simulink model "Marine_LocoMotive_UAV"  (R2018a)
settings: Solver=ode4  StartTime=0.0  StopTime=60  FixedStep=T  RelTol=1e-3
values from neighbouring files (symbols this model uses):
  a_11 = 0.05*m_b    (= 0.625)    [Marine_LocoMotive_UAV_parameters.m]
  a_33 = m_b    (= 12.5)    [Marine_LocoMotive_UAV_parameters.m]
  A_w = 1*1.5/2    (= 0.75)    [Marine_LocoMotive_UAV_parameters.m]
  A_w2 = 1*0.27/2    (= 0.135)    [Marine_LocoMotive_UAV_parameters.m]
  alpha_bar = pi/4    (= 0.785398163397)    [Marine_LocoMotive_UAV_parameters.m]
  Am = sysd.denominator{1}    [Marine_LocoMotive_UAV_parameters.m]
  Am1_LPF = sysd.denominator{1}    [Marine_LocoMotive_UAV_parameters.m]
  Am2_LPF = sysd.denominator{1}    [Marine_LocoMotive_UAV_parameters.m]
  AmAlpha_LPF = sysd.denominator{1}    [Marine_LocoMotive_UAV_parameters.m]
  AmV_LPF = sysd.denominator{1}    [Marine_LocoMotive_UAV_parameters.m]
  AmZ_LPF = sysd.denominator{1}    [Marine_LocoMotive_UAV_parameters.m]
  b_11 = 0    [Marine_LocoMotive_UAV_parameters.m]
  b_33 = 2*m_b*omega_h    (= 27.5578302946)    [Marine_LocoMotive_UAV_parameters.m]
  Bm = sysd.numerator{1}    [Marine_LocoMotive_UAV_parameters.m]
  Bm1_LPF = sysd.numerator{1}    [Marine_LocoMotive_UAV_parameters.m]
  Bm2_LPF = sysd.numerator{1}    [Marine_LocoMotive_UAV_parameters.m]
  BmAlpha_LPF = sysd.numerator{1}    [Marine_LocoMotive_UAV_parameters.m]
  BmV_LPF = sysd.numerator{1}    [Marine_LocoMotive_UAV_parameters.m]
  BmZ_LPF = sysd.numerator{1}    [Marine_LocoMotive_UAV_parameters.m]
  C_S = [5;9]*10^-3    [Marine_LocoMotive_UAV_parameters.m]
  D_x = b_11 + D_s(1)    [Marine_LocoMotive_UAV_parameters.m]
  D_z = b_33 + D_s(2)    [Marine_LocoMotive_UAV_parameters.m]
  dc_M_p = 6.7    [Marine_LocoMotive_UAV_parameters.m]
  Delta_h = (A_im/A_b-0.5)*h_b    (= -0.0625)    [Marine_LocoMotive_UAV_parameters.m]
  epsilon_1 = 5    [Marine_LocoMotive_UAV_parameters.m]
  epsilon_w = 0    [Marine_LocoMotive_UAV_parameters.m]
  epsilon_w2 = pi    (= 3.14159265359)    [Marine_LocoMotive_UAV_parameters.m]
  g = 9.81    [Marine_LocoMotive_UAV_parameters.m]
  gamma_d_p = 2*0.3/0.03*2*0.2*12/4    (= 24)    [Marine_LocoMotive_UAV_parameters.m]
  H = 10    [Marine_LocoMotive_UAV_parameters.m]
  h_b = 0.25    [Marine_LocoMotive_UAV_parameters.m]
  J_a = m_u*Lc_0^2 + (m_u*(Lc_0/2)^2+m_u*Lc_0/12)    (= 111.3)    [Marine_LocoMotive_UAV_parameters.m]
  J_b = m_b*h_b*l_b/12    (= 0.208333333333)    [Marine_LocoMotive_UAV_parameters.m]
  J_u = 0.03    [Marine_LocoMotive_UAV_parameters.m]
  K = 20    [Marine_LocoMotive_UAV_parameters.m]
  k3 = 4.5    [Marine_LocoMotive_UAV_parameters.m]
  k4 = 2    [Marine_LocoMotive_UAV_parameters.m]
  k_w = omega_w^2/g    (= 0.123862835563)    [Marine_LocoMotive_UAV_parameters.m]
  k_w2 = omega_w2^2/g    (= 0.447144836384)    [Marine_LocoMotive_UAV_parameters.m]
  kd_a = 7    [Marine_LocoMotive_UAV_parameters.m]
  kd_t = 6    [Marine_LocoMotive_UAV_parameters.m]
  kd_T = 0.3    [Marine_LocoMotive_UAV_parameters.m]
  kd_x = 5    [Marine_LocoMotive_UAV_parameters.m]
  kd_z = 2    [Marine_LocoMotive_UAV_parameters.m]
  ki_a = 2    [Marine_LocoMotive_UAV_parameters.m]
  ki_T = 0.8    [Marine_LocoMotive_UAV_parameters.m]
  ki_x = 1.2    [Marine_LocoMotive_UAV_parameters.m]
  ki_z = 1    [Marine_LocoMotive_UAV_parameters.m]
  kp_a = 7    [Marine_LocoMotive_UAV_parameters.m]
  kp_t = 10    [Marine_LocoMotive_UAV_parameters.m]
  kp_T = 5    [Marine_LocoMotive_UAV_parameters.m]
  kp_x = 7    [Marine_LocoMotive_UAV_parameters.m]
  kp_z = 3    [Marine_LocoMotive_UAV_parameters.m]
  L = 0.2    [Marine_LocoMotive_UAV_parameters.m]
  l_b = 0.8    [Marine_LocoMotive_UAV_parameters.m]
  Lc_0 = 7    [Marine_LocoMotive_UAV_parameters.m]
  LIMIT_CMD_PITCH = 45*pi/180    (= 0.785398163397)    [Marine_LocoMotive_UAV_parameters.m]
  LIMIT_uCMD_HEIGHT = 3.5*K    (= 70)    [Marine_LocoMotive_UAV_parameters.m]
  M_a = m_u*Lc_0 + m_c*Lc_0    (= 16.1)    [Marine_LocoMotive_UAV_parameters.m]
  m_b = rho_w*Vol_b/4    (= 12.5)    [Marine_LocoMotive_UAV_parameters.m]
  m_c = 0.5    [Marine_LocoMotive_UAV_parameters.m]
  m_u = 1.8    [Marine_LocoMotive_UAV_parameters.m]
  nu_w = 1.787*10^-6    (= 1.787e-06)    [Marine_LocoMotive_UAV_parameters.m]
  omega_w = 2*pi/T_w    (= 1.10231321179)    [Marine_LocoMotive_UAV_parameters.m]
  omega_w2 = 2*pi/T_w2    (= 2.09439510239)    [Marine_LocoMotive_UAV_parameters.m]
  rho_w = 1000    [Marine_LocoMotive_UAV_parameters.m]
  T = 1/100    (= 0.01)    [Marine_LocoMotive_UAV_parameters.m]
  Theta0 = atan2(V_bar*D_x*cos(alpha_bar_0),V_bar*D_x*sin(alpha_bar_0)+m_u*g*cos(alpha_bar_0))    [Marine_LocoMotive_UAV_parameters.m]
  u_s = w_dir*A_w^2*omega_w*k_w*exp(2*k_w*(-Delta_h/2))    [Marine_LocoMotive_UAV_parameters.m]
  u_s2 = w_dir2*A_w2^2*omega_w2*k_w2*exp(2*k_w2*(-Delta_h/2))    [Marine_LocoMotive_UAV_parameters.m]
  u_t = 0*0.2*1    (= 0)    [Marine_LocoMotive_UAV_parameters.m]
  u_w = 0*0.2    (= 0)    [Marine_LocoMotive_UAV_parameters.m]
  V0_b = [u_t+u_w+u_s+u_s2+v_x_w, v_z_w]    [Marine_LocoMotive_UAV_parameters.m]
  V_bar = 5    [Marine_LocoMotive_UAV_parameters.m]
  Vol_b = A_b*l_b    (= 0.05)    [Marine_LocoMotive_UAV_parameters.m]
  w_dir = 1    [Marine_LocoMotive_UAV_parameters.m]
  w_dir2 = 1    [Marine_LocoMotive_UAV_parameters.m]
  X0_b = [0,H+Zeta_0-Delta_h]    [Marine_LocoMotive_UAV_parameters.m]
  zu_bar = X0_b(2) + Lc_0*sin(alpha_bar_0)    [Marine_LocoMotive_UAV_parameters.m]
undefined symbols (not defined in the file or in its folder): DiscIntNeverNeededParam, k_Da, k_Pa, R_b, Zg
libraries: simulink x30, simulink_extras x3
(part 1 of 3)
settings Model: Creator=Ahmad  LastModifiedBy=Ahmad

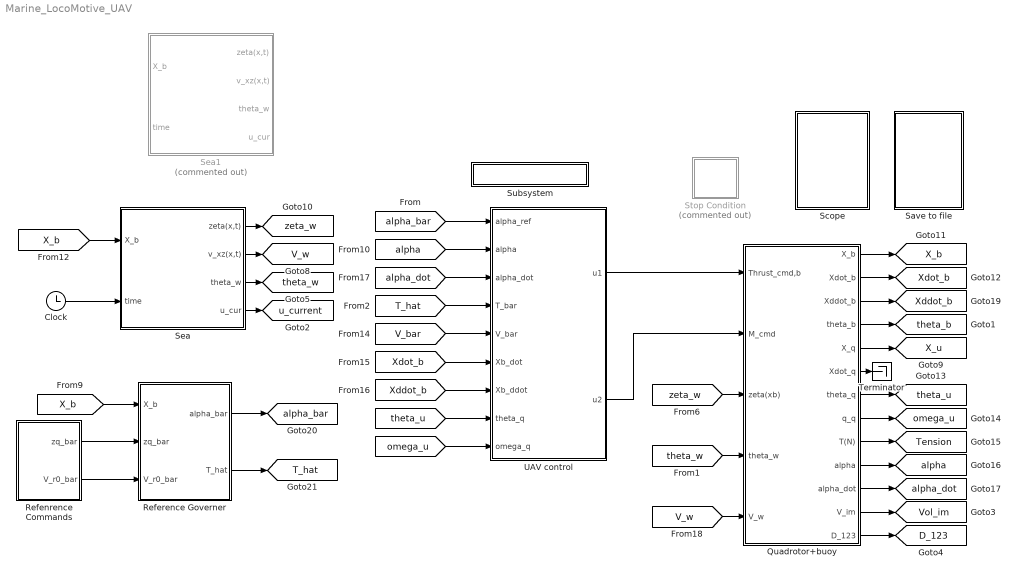
== system Marine_LocoMotive_UAV ==
  Clock : Clock
  Quadrotor+buoy : Subsystem
  Refenrence Commands : Subsystem
  Reference Governer : Subsystem
  Save to file : Subsystem
  Scope : Subsystem
  Sea : Subsystem
  Sea1 : Subsystem  Commented=on
  Stop Condition : Subsystem  Commented=on
  Subsystem : Subsystem
      settings: OpenFcn=Marine_LocoMotive_UAV_parameters
      mask Display:
      | text(.5,.5,'load parameters',...
      | 	'horizontalalignment','center');
  Terminator : Terminator
  UAV control : Subsystem
  tag scope: D_123=global, T_hat=global, Tension=global, V_w=global, Vol_im=global, X_b=global, X_u=global, Xddot_b=global, Xdot_b=global, alpha=global, alpha_bar=global, alpha_dot=global, omega_u=global, theta_b=global, theta_u=global, theta_w=global, u_current=global, zeta_w=global
  wires:
  Clock/1 -> Sea/2(time)
  [X_b] -> Sea/1(X_b)
  Sea/1(zeta(x,t)) -> [zeta_w]
  Sea/2(v_xz(x,t)) -> [V_w]
  Sea/3(theta_w) -> [theta_w]
  [theta_w] -> Quadrotor+buoy/4(theta_w)
  [V_w] -> Quadrotor+buoy/5(V_w)
  [zeta_w] -> Quadrotor+buoy/3(zeta(xb))
  Quadrotor+buoy/5(X_q) -> [X_u]
  Quadrotor+buoy/1(X_b) -> [X_b]
  UAV control/1(u1) -> Quadrotor+buoy/1(Thrust_cmd,b)
  UAV control/2(u2) -> Quadrotor+buoy/2(M_cmd)
  Quadrotor+buoy/2(Xdot_b) -> [Xdot_b]
  Quadrotor+buoy/7(theta_q) -> [theta_u]
  Quadrotor+buoy/8(q_q) -> [omega_u]
  Quadrotor+buoy/9(T(N)) -> [Tension]
  Quadrotor+buoy/10(alpha) -> [alpha]
  Quadrotor+buoy/11(alpha_dot) -> [alpha_dot]
  [X_b] -> Reference Governer/1(X_b)
  Refenrence Commands/1(zq_bar) -> Reference Governer/2(zq_bar)
  Reference Governer/1(alpha_bar) -> [alpha_bar]
  Reference Governer/2(T_hat) -> [T_hat]
  Quadrotor+buoy/3(Xddot_b) -> [Xddot_b]
  Refenrence Commands/2(V_r0_bar) -> Reference Governer/3(V_r0_bar)
  Quadrotor+buoy/4(theta_b) -> [theta_b]
  Quadrotor+buoy/6(Xdot_q) -> Terminator/1
  Sea/4(u_cur) -> [u_current]
  Quadrotor+buoy/12(V_im) -> [Vol_im]
  Quadrotor+buoy/13(D_123) -> [D_123]
  [alpha_bar] -> UAV control/1(alpha_ref)
  [alpha] -> UAV control/2(alpha)
  [alpha_dot] -> UAV control/3(alpha_dot)
  [T_hat] -> UAV control/4(T_bar)
  [V_bar] -> UAV control/5(V_bar)
  [Xdot_b] -> UAV control/6(Xb_dot)
  [Xddot_b] -> UAV control/7(Xb_ddot)
  [theta_u] -> UAV control/8(theta_q)
  [omega_u] -> UAV control/9(omega_q)

== system Marine_LocoMotive_UAV/Quadrotor+buoy ==
  Thrust_cmd,b : Inport
  M_cmd : Inport  Port=2
  zeta(xb) : Inport  Port=3
  theta_w : Inport  Port=4
  V_w : Inport  Port=5
  3-DOF equations of motion Earth frame : Subsystem  mask(3DOF EoM, earth frame){pos_b_ini=X0_b, theta_b_ini=0, alpha_0=alpha_bar, v_b_ini=V0_b, theta_q_ini=Theta0, q_b_ini=0, m_u=m_u, J_u=J_u, m_b=m_b, J_b=J_b, a_ii=[a_11 a_33], b_ii=[D_x,D_z], L=Lc_0, g=g}
      mask prompts: pos_b_ini "Buoy initial position (x z):"; theta_b_ini "Buoy initial body attitude (quadrotor):"; alpha_0 "Cable initial angle:"; v_b_ini "Buoy initial velocity (buoy):"; theta_q_ini "Quadrotor initial body attitude (quadrotor):"; q_b_ini "Quadrotor initial body rotation rate:"; m_u "Quadrotor mass:"; J_u "Quadrotor moment of Inertia:"; m_b "Buoy mass:"; J_b "Buoy moment of Inertia:"; a_ii "Added mass (1x3):"; b_ii "Buoy damping coefficients (1x2):"; L "Cable length:"; g "gravity:"
      mask Display:
      | port_label('input',1,'u_1 (N)','texmode','on');
      | port_label('input',2,'u_2 (N.m)','texmode','on');
      | port_label('input',3,'\zeta (m)','texmode','on');
      | port_label('input',4,'\theta_w (rad)','texmode','on');
      | port_label('input',5,'V_w (N.mm/s)','texmode','on');
      | 
      | port_label('output',1,'X_b (m)','texmode','on');
      | port_label('output',2,'X_{b,dot} (m/s)','texmode','on');
      | port_label('output',3,'X_{b,ddot} (m/s)','texmode','on');
      | port_label('output',4,'\theta_b(rad)','texmode','on');
      | port_label('output',5,'X_q (m)','texmode','on');
      | port_label('output',6,'X_{q,dot} (m/s)','texmode','on');
      | port_label('output',7,'\theta_q(rad)','texmode','on');
      | port_label('output',8,'\omega_q (rad/s)','texmode','on');
      | port_label('output',9,'\alpha (rad)','texmode','on');
      | port_label('output',10,'\alpha_{dot} (rad/s)','texmode','on');
      | port_label('output',11,'T (N)','texmode','on');
      | port_label('output',12,'V_{im} (m^3)','texmode','on');
      | port_label('output',13,'D_{123}','texmode','on');
  Gain : Gain
  Gain1 : Gain
  Mux : Mux  Inputs=2
  Mux1 : Mux  Inputs=2
  Saturation - Limit Height Controller1 : Saturate  UpperLimit=K*L*1.41  LowerLimit=-K*L*1.41
  Saturation - Limit Height Controller3 : Saturate  UpperLimit=4*K  LowerLimit=0
  Torque : Scope
  "Xb " : Scope
  "Xq " : Scope
  motor dynamics (thrust) : DiscreteTransferFcn  Numerator=Bm  Denominator=Am  InitialStates=-Am(2)/Bm(2)*m_u*g/cos(Theta0)
  motor dynamics (torque) : DiscreteTransferFcn  Numerator=Bm  Denominator=Am
  thrust : Scope
  X_b : Outport
  Xdot_b : Outport  Port=2
  Xddot_b : Outport  Port=3
  theta_b : Outport  Port=4
  X_q : Outport  Port=5
  Xdot_q : Outport  Port=6
  theta_q : Outport  Port=7
  q_q : Outport  Port=8
  T(N) : Outport  Port=9
  alpha : Outport  Port=10
  alpha_dot : Outport  Port=11
  V_im : Outport  Port=12
  D_123 : Outport  Port=13
  wires:
  Saturation - Limit Height Controller3/1 -> Gain/1, Mux/2
  motor dynamics (torque)/1 -> Saturation - Limit Height Controller1/1
  M_cmd/1 -> Mux1/1, motor dynamics (torque)/1
  Thrust_cmd,b/1 -> Mux/1, motor dynamics (thrust)/1
  Saturation - Limit Height Controller1/1 -> Mux1/2, Gain1/1
  zeta(xb)/1 -> 3-DOF equations of motion Earth frame/3(zeta)
  theta_w/1 -> 3-DOF equations of motion Earth frame/4(theta_w)
  V_w/1 -> 3-DOF equations of motion Earth frame/5(V_w)
  3-DOF equations of motion Earth frame/5(Xu) -> "Xq "/1, X_q/1  "X_q"
  3-DOF equations of motion Earth frame/1(Xb) -> "Xb "/1, X_b/1  "X_b"
  3-DOF equations of motion Earth frame/2(Xb_dot) -> Xdot_b/1  "Xdot_b"
  3-DOF equations of motion Earth frame/6(Xu_dot) -> Xdot_q/1  "V_q"
  3-DOF equations of motion Earth frame/4(Attitude_buoy) -> theta_b/1  "theta_b"
  3-DOF equations of motion Earth frame/7(Attitude_quadrotor) -> theta_q/1  "theta_q"
  3-DOF equations of motion Earth frame/8(q_quadrotor) -> q_q/1  "omega_q"
  3-DOF equations of motion Earth frame/3(Xb_ddot) -> Xddot_b/1
  motor dynamics (thrust)/1 -> Saturation - Limit Height Controller3/1
  3-DOF equations of motion Earth frame/10(alpha_dot) -> alpha_dot/1  "alpha_dot"
  3-DOF equations of motion Earth frame/11(Cable Tension) -> T(N)/1  "tension"
  3-DOF equations of motion Earth frame/9(alpha) -> alpha/1  "alpha"
  Mux/1 -> thrust/1
  Mux1/1 -> Torque/1
  3-DOF equations of motion Earth frame/12(V_im) -> V_im/1
  Gain/1 -> 3-DOF equations of motion Earth frame/1(u1)
  Gain1/1 -> 3-DOF equations of motion Earth frame/2(u2)
  3-DOF equations of motion Earth frame/13("D_123 ") -> D_123/1

== system Marine_LocoMotive_UAV/Refenrence Commands ==
  note: V_r0_bar is the velocity of the buoy relative
      | to the water current (wave velocity is not included)
  note: Refecence velocity
  "Bias1 " : Bias  Bias=u_t+u_w+u_s
  Bias1 1 : Bias  Commented=on  Bias=u_t+u_w+u_s
  Bias2 : Bias  Bias=-(u_t+u_w+u_s+u_s2)
  Discrete Transfer Fcn : DiscreteTransferFcn  Numerator=BmV_LPF  Denominator=AmV_LPF  InitialStates=sum(AmV_LPF)/sum(BmV_LPF)*0
  Manual Switch : ManualSwitch
  Measured?? (this is not real!) : From  Commented=on  GotoTag=V_w  TagVisibility=global
  Mux : Mux  Inputs=2
  Ramp : simulink/Sources/Ramp  Commented=on  slope=10/40  start=0  InitialOutput=0
  Rate Limiter : RateLimiter  Commented=on  RisingSlewLimit=1/4  FallingSlewLimit=-1/4  SampleTimeMode=inherited
  Step : Step  Time=0  After=V_bar  SampleTime=0
  Step1 : Step  Time=30  After=2  SampleTime=0
  Sum : Sum  Inputs=|+-
  Sum1 : Sum  Inputs=|+-
  V_bar (desired Velocity) : Scope
  v_x : Selector  Commented=on  InputPortWidth=2  IndexOptions=Index vector (dialog)  Indices=[1]  OutputSizes=1
  z_dez : Constant  Value=zu_bar
  zq_bar : Outport
  V_r0_bar : Outport  Port=2
  tag scope: V_bar=global, V_r_bar=global, z_bar=global
  wires:
  Step/1 -> Sum/1
  Step1/1 -> Sum/2
  Measured?? (this is not real!)/1 -> v_x/1
  Manual Switch/1 -> Sum1/2
  Sum1/1 -> V_r0_bar/1, [V_r_bar]  "V_tilde"
  Discrete Transfer Fcn/1 -> "Bias1 "/1
  Mux/1 -> V_bar (desired Velocity)/1
  z_dez/1 -> [z_bar], zq_bar/1
  v_x/1 -> Manual Switch/2
  [u_current] -> Manual Switch/1
  Ramp/1 -> Bias1 1/1
  Bias2/1 -> Discrete Transfer Fcn/1
  Sum/1 -> Bias2/1, Mux/1
  "Bias1 "/1 -> [V_bar], Sum1/1, Mux/2

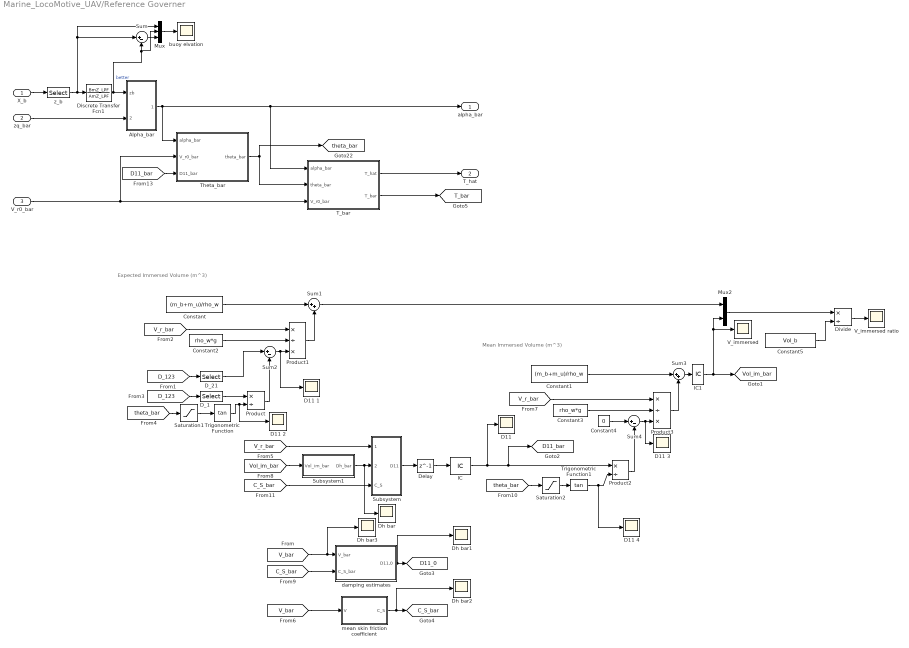
== system Marine_LocoMotive_UAV/Reference Governer ==
  note: Expected Immersed Volume (m^3)
  note: Mean Immersed Volume (m^3)
  X_b : Inport
  zq_bar : Inport  Port=2
  V_r0_bar : Inport  Port=3
  Alpha_bar : Subsystem
  Constant : Constant  Value=(m_b+m_u)/rho_w
  Constant1 : Constant  Value=(m_b+m_u)/rho_w
  Constant2 : Constant  Value=rho_w*g
  Constant3 : Constant  Value=rho_w*g
  Constant4 : Constant  Value=0
  Constant5 : Constant  Value=Vol_b
  D11 {,1..4} (5 alike) : Scope
  D_1 : Selector  NumberOfDimensions=2  InputPortWidth=2  IndexOptions=Index vector (dialog),Index vector (dialog)  Indices=1,1  OutputSizes=1,1
  D_21 : Selector  NumberOfDimensions=2  InputPortWidth=2  IndexOptions=Index vector (dialog),Index vector (dialog)  Indices=2,1  OutputSizes=1,1
  Delay : Delay  DelayLength=1  InitialCondition=0
  Dh bar{,1..3} (4 alike) : Scope
  Discrete Transfer Fcn1 : DiscreteTransferFcn  Numerator=BmZ_LPF  Denominator=AmZ_LPF  InitialStates=[1 1]*(1-sum(AmZ_LPF))/(sum(BmZ_LPF))*X0_b(2)
  Divide : Product  Inputs=*/
  IC : InitialCondition  Value=D_x
  IC1 : InitialCondition  Value=Delta_h*l_b*h_b + l_b*h_b^2/2
  Mux : Mux  Inputs=3
  Mux2 : Mux  Inputs=2
  Product : Product  Inputs=*/
  Product1 : Product  Inputs=*/*
  Product2 : Product  Inputs=*/
  Product3 : Product  Inputs=*/*
  Saturation1 : Saturate  UpperLimit=inf  LowerLimit=0.1*pi/180
  Saturation2 : Saturate  UpperLimit=inf  LowerLimit=0.1*pi/180
  Subsystem : Subsystem
  Subsystem1 : Subsystem
  Sum : Sum  Inputs=|+-
  Sum1 : Sum  Inputs=|++
  Sum2 : Sum  Inputs=|+-
  Sum3 : Sum  Inputs=|++
  Sum4 : Sum  Inputs=|+-
  "T_bar " : Subsystem
  "Theta_bar " : Subsystem
  Trigonometric Function : Trigonometry  Operator=tan
  Trigonometric Function1 : Trigonometry  Operator=tan
  V_immersed : Scope
  V_immersed ratio : Scope
  buoy elvation : Scope
  damping estimates : Subsystem
  "mean skin friction coefficient " : Subsystem
  z_b : Selector  InputPortWidth=2  IndexOptions=Index vector (dialog)  Indices=2  OutputSizes=1
  alpha_bar : Outport
  T_hat : Outport  Port=2
  tag scope: C_S_bar=global, D11_0=global, D11_bar=global, T_bar=global, Vol_im_bar=global, theta_bar=global
  wires:
  X_b/1 -> z_b/1
  "Theta_bar "/1(theta_bar) -> [theta_bar], "T_bar "/2(theta_bar)
  V_r0_bar/1 -> "Theta_bar "/2(V_r0_bar), "T_bar "/3(V_r0_bar)
  zq_bar/1 -> Alpha_bar/2(zq_bar)
  Mux/1 -> buoy elvation/1
  Sum/1 -> Mux/3
  Trigonometric Function/1 -> D11 2/1, Product/2
  Sum1/1 -> Mux2/1
  [theta_bar] -> Saturation1/1
  [D_123] -> D_21/1
  Constant/1 -> Sum1/1
  [V_r_bar] -> Product1/1
  Constant2/1 -> Product1/2
  Product1/1 -> Sum1/2
  Sum2/1 -> D11 1/1, Product1/3
  [D_123] -> D_1/1
  D_21/1 -> Sum2/1
  Product/1 -> Sum2/2
  D_1/1 -> Product/1
  [V_r_bar] -> Subsystem/1(Vr_bar)
  Subsystem1/1(Dh_bar) -> Dh bar/1, Subsystem/2(Dh_bar)
  [Vol_im_bar] -> Subsystem1/1(Vol_im_bar)
  IC/1 -> "D11 "/1, Product2/1, [D11_bar]
  Product2/1 -> Sum4/2
  Constant4/1 -> Sum4/1
  Subsystem/1(D11) -> Delay/1
  Sum4/1 -> D11 3/1, Product3/3
  Product3/1 -> Sum3/2
  Constant3/1 -> Product3/2
  [V_r_bar] -> Product3/1
  Constant1/1 -> Sum3/1
  [theta_bar] -> Saturation2/1
  Trigonometric Function1/1 -> D11 4/1, Product2/2
  Mux2/1 -> Divide/1
  IC1/1 -> V_immersed/1, Mux2/2, [Vol_im_bar]
  Delay/1 -> IC/1
  Sum3/1 -> IC1/1
  Constant5/1 -> Divide/2
  Divide/1 -> V_immersed ratio/1
  z_b/1 -> Discrete Transfer Fcn1/1, Sum/1, Mux/1
  Discrete Transfer Fcn1/1 -> Mux/2, Sum/2, Alpha_bar/1(zb)  "better"
  [V_bar] -> Dh bar3/1, damping estimates/1(V_bar)
  damping estimates/1(D11,0) -> Dh bar1/1, [D11_0]
  [C_S_bar] -> damping estimates/2(C_S_bar)
  [V_bar] -> "mean skin friction coefficient "/1(V)
  [C_S_bar] -> Subsystem/3(C_S)
  "mean skin friction coefficient "/1(C_S) -> Dh bar2/1, [C_S_bar]
  Saturation1/1 -> Trigonometric Function/1
  Saturation2/1 -> Trigonometric Function1/1
  [D11_bar] -> "Theta_bar "/3(D11_bar)
  Alpha_bar/1(alpha_bar) -> alpha_bar/1, "T_bar "/1("alpha_bar "), "Theta_bar "/1("alpha_bar ")
  "T_bar "/1(T_hat) -> T_hat/1
  "T_bar "/2(T_bar) -> [T_bar]

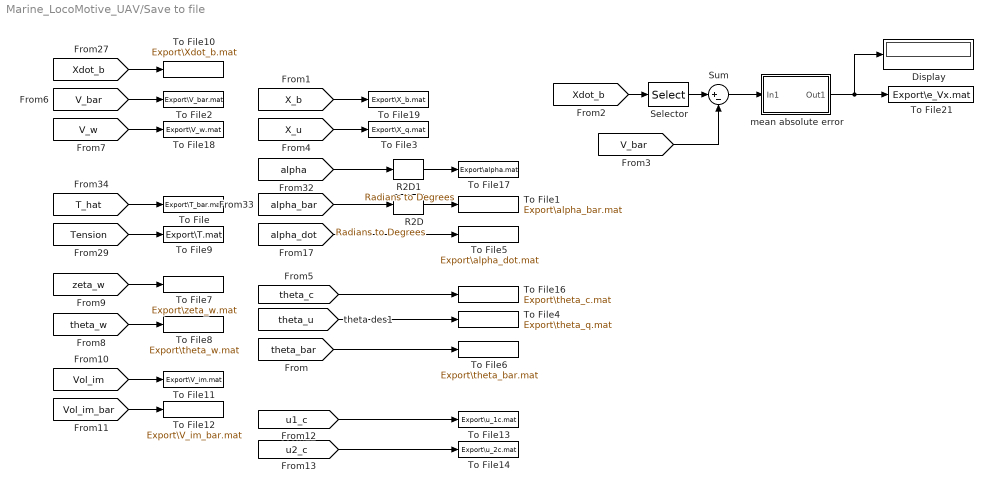
== system Marine_LocoMotive_UAV/Save to file ==
  Display : Display
  R2D : simulink_extras/Transformations/Radians to Degrees
  R2D1 : simulink_extras/Transformations/Radians to Degrees
  Selector : Selector  InputPortWidth=2  IndexOptions=Index vector (dialog)  Indices=1  OutputSizes=1
  Sum : Sum  Inputs=|+-
  To File : ToFile  Filename=Export\T_bar.mat  MatrixName=T_bar  SaveFormat=Timeseries  SampleTime=floor(T/4)
  To File1 : ToFile  Filename=Export\alpha_bar.mat  MatrixName=alpha_bar  SaveFormat=Timeseries  SampleTime=floor(T/4)
  To File10 : ToFile  Filename=Export\Xdot_b.mat  MatrixName=Xdot_b  SaveFormat=Timeseries  SampleTime=floor(T/4)
  To File11 : ToFile  Filename=Export\V_im.mat  MatrixName=V_im  SaveFormat=Timeseries  SampleTime=floor(T/4)
  To File12 : ToFile  Filename=Export\V_im_bar.mat  MatrixName=V_im_bar  SaveFormat=Timeseries  SampleTime=floor(T/4)
  To File13 : ToFile  Filename=Export\u_1c.mat  MatrixName=u_1c  SaveFormat=Timeseries  SampleTime=floor(T/4)
  To File14 : ToFile  Filename=Export\u_2c.mat  MatrixName=u_2c  SaveFormat=Timeseries  SampleTime=floor(T/4)
  To File16 : ToFile  Filename=Export\theta_c.mat  MatrixName=theta_c  SaveFormat=Timeseries  SampleTime=floor(T/4)
  To File17 : ToFile  Filename=Export\alpha.mat  MatrixName=alpha  SaveFormat=Timeseries  SampleTime=floor(T/4)
  To File18 : ToFile  Filename=Export\V_w.mat  MatrixName=V_w  SaveFormat=Timeseries  SampleTime=floor(T/4)
  To File19 : ToFile  Filename=Export\X_b.mat  MatrixName=X_b  SaveFormat=Timeseries  SampleTime=floor(T/4)
  To File2 : ToFile  Filename=Export\V_bar.mat  MatrixName=V_bar  SaveFormat=Timeseries  SampleTime=floor(T/4)
  To File21 : ToFile  Filename=Export\e_Vx.mat  MatrixName=Vx  SaveFormat=Timeseries  SampleTime=floor(T/4)
  To File3 : ToFile  Filename=Export\X_q.mat  MatrixName=X_q  SaveFormat=Timeseries  SampleTime=floor(T/4)
  To File4 : ToFile  Filename=Export\theta_q.mat  MatrixName=theta_q  SaveFormat=Timeseries  SampleTime=floor(T/4)
  To File5 : ToFile  Filename=Export\alpha_dot.mat  MatrixName=alpha_dot  SaveFormat=Timeseries  SampleTime=floor(T/4)
  To File6 : ToFile  Filename=Export\theta_bar.mat  MatrixName=theta_bar  SaveFormat=Timeseries  SampleTime=floor(T/4)
  To File7 : ToFile  Filename=Export\zeta_w.mat  MatrixName=zeta_w  SaveFormat=Timeseries  SampleTime=floor(T/4)
  To File8 : ToFile  Filename=Export\theta_w.mat  MatrixName=theta_w  SaveFormat=Timeseries  SampleTime=floor(T/4)
  To File9 : ToFile  Filename=Export\T.mat  MatrixName=T  SaveFormat=Timeseries  SampleTime=floor(T/4)
  mean absolute error : Subsystem
  wires:
  R2D/1 -> To File1/1
  [X_u] -> To File3/1
  [alpha_bar] -> R2D/1
  [V_bar] -> To File2/1
  [theta_c] -> To File16/1
  [alpha] -> R2D1/1
  R2D1/1 -> To File17/1
  [V_w] -> To File18/1
  [X_b] -> To File19/1
  Sum/1 -> mean absolute error/1(In1)
  mean absolute error/1(Out1) -> Display/1, To File21/1
  [T_hat] -> To File/1
  [theta_u] -> To File4/1
  [alpha_dot] -> To File5/1
  [theta_bar] -> To File6/1
  [zeta_w] -> To File7/1
  [theta_w] -> To File8/1
  [Tension] -> To File9/1
  [Xdot_b] -> To File10/1
  [Xdot_b] -> Selector/1
  [V_bar] -> Sum/2
  Selector/1 -> Sum/1
  [Vol_im] -> To File11/1
  [Vol_im_bar] -> To File12/1
  [u1_c] -> To File13/1
  [u2_c] -> To File14/1

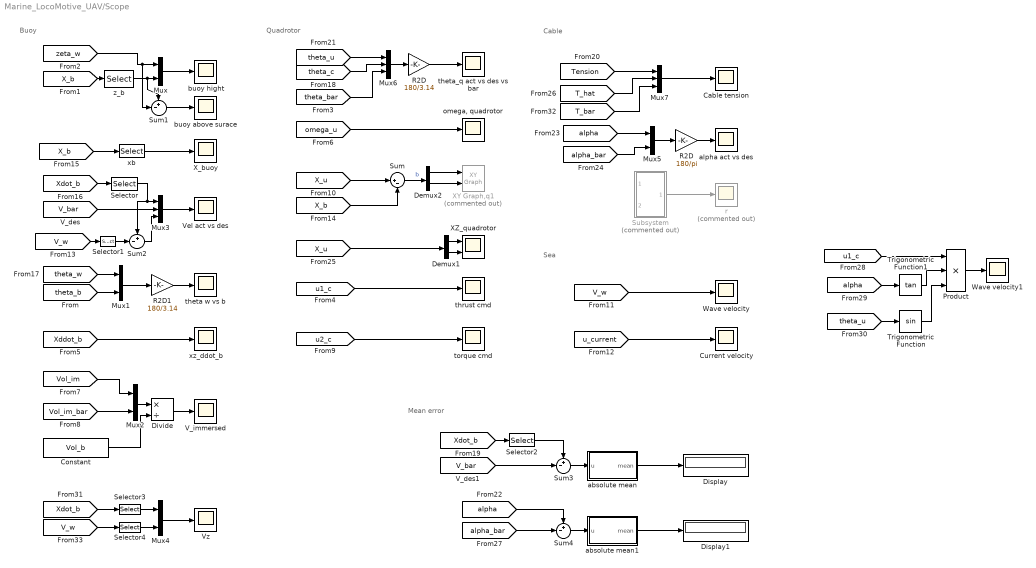
== system Marine_LocoMotive_UAV/Scope ==
  note: Mean error
  note: Sea
  note: Cable
  note: Quadrotor
  note: Buoy
  Cable tension : Scope
  Constant : Constant  Value=Vol_b
  Current velocity : Scope
  Demux1 : Demux  Outputs=2
  Demux2 : Demux  Outputs=2
  Display : Display
  Display1 : Display
  Divide : Product  Inputs=*/
  Mux{,1..2,4..5} (5 alike) : Mux  Inputs=2
  Mux3 : Mux  Inputs=3
  Mux6 : Mux  Inputs=3
  Mux7 : Mux  Inputs=3
  Product : Product  Inputs=3
  R2D : Gain  Gain=180/3.14
  "R2D " : Gain  Gain=180/pi
  R2D1 : Gain  Gain=180/3.14
  Selector : Selector  InputPortWidth=2  IndexOptions=Index vector (dialog)  Indices=1  OutputSizes=1
  Selector1 : Selector  InputPortWidth=2  IndexOptions=Index vector (dialog)  Indices=1  OutputSizes=1
  Selector2 : Selector  InputPortWidth=2  IndexOptions=Index vector (dialog)  Indices=1  OutputSizes=1
  Selector3 : Selector  InputPortWidth=2  IndexOptions=Index vector (dialog)  Indices=2  OutputSizes=1
  Selector4 : Selector  InputPortWidth=2  IndexOptions=Index vector (dialog)  Indices=2  OutputSizes=1
  Subsystem : Subsystem  Commented=on
  Sum : Sum  Inputs=|+-
  Sum{1..4} (4 alike) : Sum  Inputs=+-|
  Trigonometric Function : Trigonometry
  Trigonometric Function1 : Trigonometry  Operator=tan
  V_immersed : Scope
  Vel act vs des : Scope
  Vz : Scope
  Wave velocity : Scope
  Wave velocity1 : Scope
  XY Graph,q1 : simulink/Sinks/XY Graph  Commented=on  xmin=0  xmax=5  ymin=0  ymax=5  st=1/250
  XZ_quadrotor : Scope  NumInputPorts=2
  X_buoy : Scope
  absolute mean : Subsystem
  absolute mean1 : Subsystem
  "alpha act vs des " : Scope
  buoy above surace : Scope
  buoy hight : Scope
  "omega, quadrotor" : Scope
  r : Scope  Commented=on
  theta w vs b : Scope
  theta_q act vs des vs bar : Scope
  thrust cmd : Scope
  torque cmd : Scope
  xb : Selector  InputPortWidth=2  IndexOptions=Index vector (dialog)  Indices=1  OutputSizes=1
  xz_ddot_b : Scope
  z_b : Selector  InputPortWidth=2  IndexOptions=Index vector (dialog)  Indices=2  OutputSizes=1
  wires:
  Mux/1 -> buoy hight/1
  z_b/1 -> Sum1/1, Mux/2
  [zeta_w] -> Sum1/2, Mux/1
  [omega_u] -> "omega, quadrotor"/1
  [X_b] -> Sum/2
  Sum/1 -> Demux2/1  "b"
  [X_b] -> z_b/1
  Sum1/1 -> buoy above surace/1
  Mux1/1 -> R2D1/1
  Mux6/1 -> R2D/1
  Mux7/1 -> Cable tension/1
  Demux2/2 -> XY Graph,q1/2
  Demux2/1 -> XY Graph,q1/1
  [V_bar] -> Mux3/2
  [Xdot_b] -> Selector/1
  [theta_c] -> Mux6/2
  [theta_u] -> Mux6/1
  Mux3/1 -> Vel act vs des/1
  [alpha] -> Mux5/1
  [alpha_bar] -> Mux5/2
  Mux5/1 -> "R2D "/1
  [X_u] -> Sum/1
  [X_u] -> Demux1/1
  Selector/1 -> Sum2/1, Mux3/1
  "R2D "/1 -> "alpha act vs des "/1
  [Tension] -> Mux7/1
  [T_hat] -> Mux7/2
  [theta_b] -> Mux1/2
  [theta_w] -> Mux1/1
  Subsystem/1(Out1) -> r/1
  [theta_bar] -> Mux6/3
  R2D/1 -> theta_q act vs des vs bar/1
  [X_b] -> xb/1
  xb/1 -> X_buoy/1
  [Xddot_b] -> xz_ddot_b/1
  [Vol_im] -> Mux2/1
  [Vol_im_bar] -> Mux2/2
  Divide/1 -> V_immersed/1
  R2D1/1 -> theta w vs b/1
  Mux2/1 -> Divide/1
  Constant/1 -> Divide/2
  [u1_c] -> thrust cmd/1
  [u2_c] -> torque cmd/1
  [V_w] -> Wave velocity/1
  [u_current] -> Current velocity/1
  Demux1/2 -> XZ_quadrotor/2
  Demux1/1 -> XZ_quadrotor/1
  [V_w] -> Selector1/1
  Sum2/1 -> Mux3/3
  Selector1/1 -> Sum2/2
  [Xdot_b] -> Selector2/1
  [V_bar] -> Sum3/2
  Selector2/1 -> Sum3/1
  Sum3/1 -> absolute mean/1(u)
  absolute mean/1(mean) -> Display/1
  [alpha] -> Sum4/1
  [alpha_bar] -> Sum4/2
  Sum4/1 -> absolute mean1/1(u)
  absolute mean1/1(mean) -> Display1/1
  [alpha] -> Trigonometric Function1/1
  [theta_u] -> Trigonometric Function/1
  [u1_c] -> Product/1
  Trigonometric Function1/1 -> Product/2
  Trigonometric Function/1 -> Product/3
  Product/1 -> Wave velocity1/1
  [T_bar] -> Mux7/3
  [Xdot_b] -> Selector3/1
  [V_w] -> Selector4/1
  Selector4/1 -> Mux4/2
  Mux4/1 -> Vz/1
  Selector3/1 -> Mux4/1

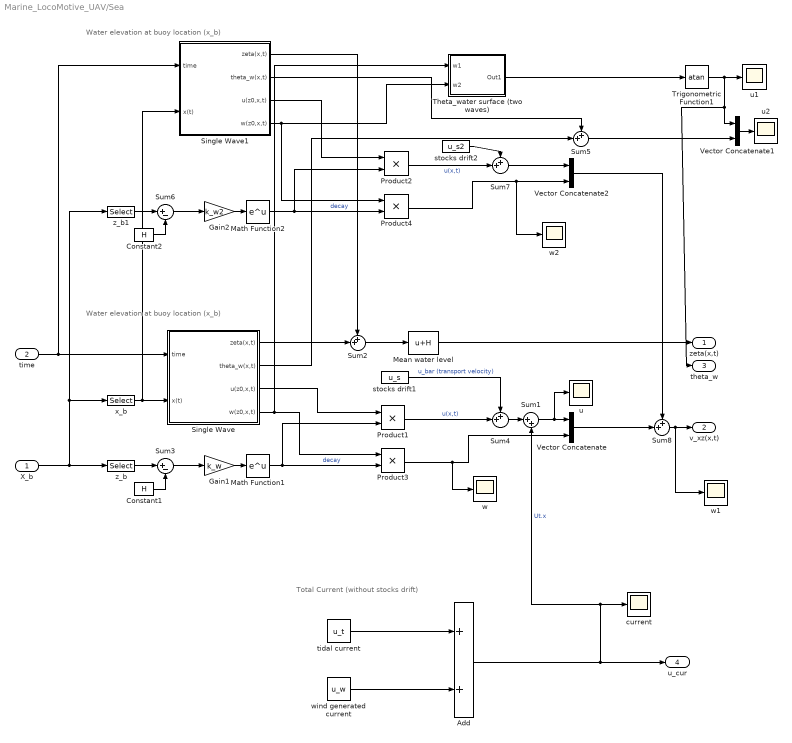
== system Marine_LocoMotive_UAV/Sea ==
  note: Water elevation at buoy location (x_b)
  note: Total Current (without stocks drift)
  note: Water elevation at buoy location (x_b)
  X_b : Inport
  time : Inport  Port=2
  " current" : Scope
  Add : Sum  Inputs=2
  Constant1 : Constant  Value=H
  Constant2 : Constant  Value=H
  Gain1 : Gain  Gain=k_w
  Gain2 : Gain  Gain=k_w2
  Math Function1 : Math  SaturateOnIntegerOverflow=on
  Math Function2 : Math  SaturateOnIntegerOverflow=on
  Mean water level : Bias  Bias=H
  Product{1..4} (4 alike) : Product
  Single Wave : Subsystem  mask(Wave Model){A=A_w, omega=omega_w, k=k_w, epsilon=epsilon_w, w_dir=w_dir}
      mask prompts: A "Wave amplitude, A (m):"; omega "Circular frequency (rad):"; k "wave number, k:"; epsilon "Random phase angle (rad):"; w_dir "Wave direction:"
      mask help: Wave Model for a single wave in 2D.
      mask Display:
      | port_label('input',1,'t (s)','texmode','on');
      | port_label('input',2,'x(t) (m)','texmode','on');
      | 
      | port_label('output',1,'\zeta (x,t)','texmode','on');
      | port_label('output',2,'\theta_{w} (x,t)','texmode','on');
      | port_label('output',3,'u(z_0,x,t) (m/s)','texmode','on');
      | port_label('output',4,'w(z_0,x,t) (m/s)','texmode','on');
  Single Wave1 : Subsystem  mask(Wave Model){A=A_w2, omega=omega_w2, k=k_w2, epsilon=epsilon_w2, w_dir=w_dir2}
      mask prompts: A "Wave amplitude, A (m):"; omega "Circular frequency (rad):"; k "wave number, k:"; epsilon "Random phase angle (rad):"; w_dir "Wave direction:"
      mask help: Wave Model for a single wave in 2D.
      mask Display:
      | port_label('input',1,'t (s)','texmode','on');
      | port_label('input',2,'x(t) (m)','texmode','on');
      | 
      | port_label('output',1,'\zeta (x,t)','texmode','on');
      | port_label('output',2,'\theta_{w} (x,t)','texmode','on');
      | port_label('output',3,'u(z_0,x,t) (m/s)','texmode','on');
      | port_label('output',4,'w(z_0,x,t) (m/s)','texmode','on');
  Sum1 : Sum  Inputs=|++
  Sum{2,4..5,7..8} (5 alike) : Sum  Inputs=++|
  Sum3 : Sum  Inputs=|+-
  Sum6 : Sum  Inputs=|+-
  Theta_water surface (two waves) : Subsystem
  Trigonometric Function1 : Trigonometry  Operator=atan
  Vector Concatenate : Concatenate
  Vector Concatenate1 : Concatenate
  Vector Concatenate2 : Concatenate
  stocks drift1 : Constant  Value=u_s
  stocks drift2 : Constant  Value=u_s2
  tidal current : Constant  Value=u_t
  u : Scope
  u1 : Scope
  u2 : Scope
  w : Scope
  w1 : Scope
  w2 : Scope
  wind generated current : Constant  Value=u_w
  x_b : Selector  InputPortWidth=2  IndexOptions=Index vector (dialog)  Indices=1  OutputSizes=1
  z_b : Selector  InputPortWidth=2  IndexOptions=Index vector (dialog)  Indices=2  OutputSizes=1
  z_b1 : Selector  InputPortWidth=2  IndexOptions=Index vector (dialog)  Indices=2  OutputSizes=1
  zeta(x,t) : Outport
  v_xz(x,t) : Outport  Port=2
  theta_w : Outport  Port=3
  u_cur : Outport  Port=4
  wires:
  z_b/1 -> Sum3/1
  tidal current/1 -> Add/1
  wind generated current/1 -> Add/2
  Sum1/1 -> u/1, Vector Concatenate/1
  Add/1 -> u_cur/1, " current"/1, Sum1/2  "Ut.x"
  Vector Concatenate/1 -> Sum8/2
  Constant1/1 -> Sum3/2
  Single Wave/2(theta_w(x,t)) -> Sum5/2
  time/1 -> Single Wave1/1(time), Single Wave/1(time)
  x_b/1 -> Single Wave1/2(x(t)), Single Wave/2(x(t))
  Sum3/1 -> Gain1/1
  stocks drift1/1 -> Sum4/1  "u_bar (transport velocity)"
  Math Function1/1 -> Product1/2, Product3/2  "decay"
  Sum4/1 -> Sum1/1
  Product1/1 -> Sum4/2  "u(x,t)"
  Gain1/1 -> Math Function1/1
  Single Wave/1(zeta(x,t)) -> Sum2/2
  Product3/1 -> w/1, Vector Concatenate/2
  Mean water level/1 -> zeta(x,t)/1
  Single Wave/3(u(z0,x,t)) -> Product1/1
  Single Wave/4(w(z0,x,t)) -> Theta_water surface (two waves)/1(w1), Product3/1
  Trigonometric Function1/1 -> Vector Concatenate1/1, theta_w/1, u1/1
  Vector Concatenate1/1 -> u2/1
  Theta_water surface (two waves)/1(Out1) -> Trigonometric Function1/1
  Single Wave1/1(zeta(x,t)) -> Sum2/1
  Single Wave1/2(theta_w(x,t)) -> Sum5/1
  Sum5/1 -> Vector Concatenate1/2
  Sum2/1 -> Mean water level/1
  Sum6/1 -> Gain2/1
  z_b1/1 -> Sum6/1
  X_b/1 -> z_b1/1, x_b/1, z_b/1
  Gain2/1 -> Math Function2/1
  Constant2/1 -> Sum6/2
  Single Wave1/4(w(z0,x,t)) -> Product4/1, Theta_water surface (two waves)/2(w2)
  Single Wave1/3(u(z0,x,t)) -> Product2/1
  Product4/1 -> w2/1, Vector Concatenate2/2
  Product2/1 -> Sum7/2  "u(x,t)"
  Math Function2/1 -> Product4/2, Product2/2  "decay"
  stocks drift2/1 -> Sum7/1
  Sum7/1 -> Vector Concatenate2/1
  Vector Concatenate2/1 -> Sum8/1
  Sum8/1 -> w1/1, v_xz(x,t)/1

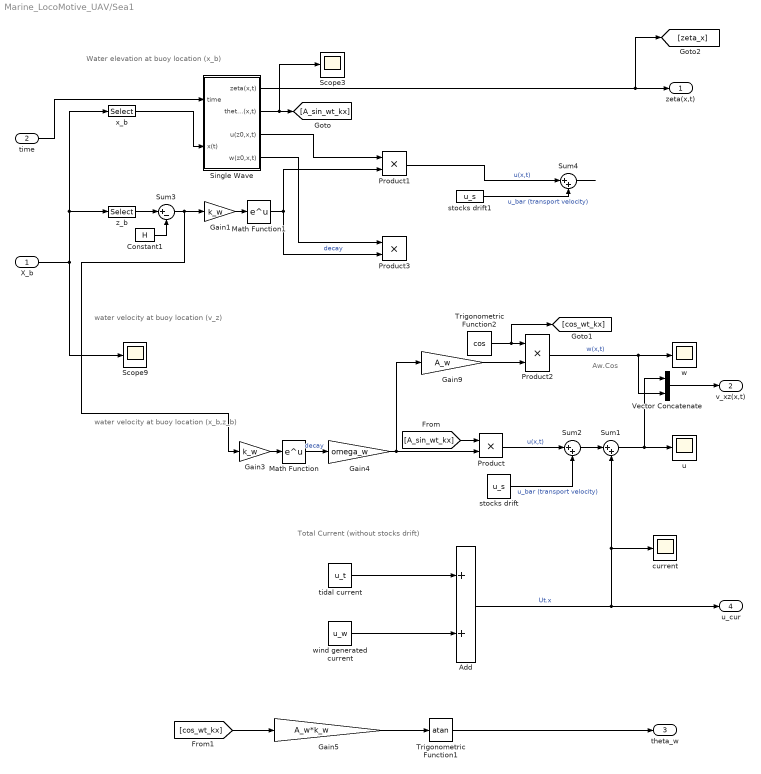
== system Marine_LocoMotive_UAV/Sea1 ==
  note: water velocity at buoy location (v_z)
  note: Total Current (without stocks drift)
  note: Water elevation at buoy location (x_b)
  note: water velocity at buoy location (x_b,z_b)
  note: Aw.Cos
  X_b : Inport
  time : Inport  Port=2
  " current" : Scope
  Add : Sum  Inputs=2
  Constant1 : Constant  Value=H
  Gain1 : Gain  Gain=k_w
  Gain3 : Gain  Gain=k_w
  Gain4 : Gain  Gain=omega_w
  Gain5 : Gain  Gain=A_w*k_w
  Gain9 : Gain  Gain=A_w
  Math Function : Math  SaturateOnIntegerOverflow=on
  Math Function1 : Math  SaturateOnIntegerOverflow=on
  Product{,1..3} (4 alike) : Product
  Scope3 : Scope
  Scope9 : Scope
  Single Wave : Subsystem
  Sum1 : Sum  Inputs=|++
  Sum2 : Sum  Inputs=|++
  Sum3 : Sum  Inputs=|+-
  Sum4 : Sum  Inputs=|++
  Trigonometric Function1 : Trigonometry  Operator=atan
  Trigonometric Function2 : Trigonometry  Operator=cos
  Vector Concatenate : Concatenate
  stocks drift : Constant  Value=u_s
  stocks drift1 : Constant  Value=u_s
  tidal current : Constant  Value=u_t
  u : Scope
  w : Scope
  wind generated current : Constant  Value=u_w
  x_b : Selector  InputPortWidth=2  IndexOptions=Index vector (dialog)  Indices=1  OutputSizes=1
  z_b : Selector  InputPortWidth=2  IndexOptions=Index vector (dialog)  Indices=2  OutputSizes=1
  zeta(x,t) : Outport
  v_xz(x,t) : Outport  Port=2
  theta_w : Outport  Port=3
  u_cur : Outport  Port=4
  wires:
  Single Wave/4(w(z0,x,t)) -> Product3/1
  Single Wave/3(u(z0,x,t)) -> Product1/1
  Gain1/1 -> Math Function1/1
  Product1/1 -> Sum4/1  "u(x,t)"
  Sum4/1 -> ?
  Math Function1/1 -> Product1/2, Product3/2  "decay"
  stocks drift1/1 -> Sum4/2  "u_bar (transport velocity)"
  Sum3/1 -> Gain1/1, Gain3/1
  x_b/1 -> Single Wave/2(x(t))
  time/1 -> Single Wave/1(time)
  Single Wave/2(theta_w(x,t)) -> [A_sin_wt_kx], Scope3/1
  Single Wave/1(zeta(x,t)) -> zeta(x,t)/1, [zeta_x]
  Constant1/1 -> Sum3/2
  Sum2/1 -> Sum1/1
  [cos_wt_kx] -> Gain5/1
  Gain5/1 -> Trigonometric Function1/1
  [A_sin_wt_kx] -> Product/1
  Vector Concatenate/1 -> v_xz(x,t)/1
  Trigonometric Function1/1 -> theta_w/1
  Gain9/1 -> Product2/2
  Trigonometric Function2/1 -> Product2/1, [cos_wt_kx]
  Gain4/1 -> Gain9/1, Product/2
  Product2/1 -> Vector Concatenate/2, w/1  "w(x,t)"
  Add/1 -> " current"/1, Sum1/2, u_cur/1  "Ut.x"
  Sum1/1 -> u/1, Vector Concatenate/1
  wind generated current/1 -> Add/2
  tidal current/1 -> Add/1
  stocks drift/1 -> Sum2/2  "u_bar (transport velocity)"
  Product/1 -> Sum2/1  "u(x,t)"
  Math Function/1 -> Gain4/1  "decay"
  z_b/1 -> Sum3/1
  X_b/1 -> Scope9/1, z_b/1, x_b/1
  Gain3/1 -> Math Function/1

== system Marine_LocoMotive_UAV/Stop Condition ==
  note: Drop Flip
  note: Crash
  note: Drained Battery
  note: Fall, landing crash
  note: Room borders crash
  Abs{,1..3} (4 alike) : Abs
  Assertion : Assertion  AssertionFailFcn=msgbox('Low Voltage!')
  Assertion1 : Assertion  AssertionFailFcn=msgbox('Crash!')
  Assertion2 : Assertion  AssertionFailFcn=msgbox('Drone Flip!')
  Compare To Constant : simulink/Logic and Bit Operations/Compare To Constant  relop=>=  const=10  OutDataTypeStr=boolean
  Compare To Constant1 : simulink/Logic and Bit Operations/Compare To Constant  relop=>=  const=10  OutDataTypeStr=boolean
  Compare To Constant2 : simulink/Logic and Bit Operations/Compare To Constant  relop=>=  const=10  OutDataTypeStr=boolean
  Compare To Constant3 : simulink/Logic and Bit Operations/Compare To Constant  relop=<=  const=Zg  OutDataTypeStr=boolean
  Compare To Constant4 : simulink/Logic and Bit Operations/Compare To Constant  relop=<  const=-1  OutDataTypeStr=boolean
  Compare To Constant5 : simulink/Logic and Bit Operations/Compare To Constant  relop=>=  const=Zg+10/100  OutDataTypeStr=boolean
  Compare To Constant6 : simulink/Logic and Bit Operations/Compare To Constant  relop=<  const=9  OutDataTypeStr=boolean
  Compare To Constant7 : simulink/Logic and Bit Operations/Compare To Constant  relop=>=  const=80  OutDataTypeStr=boolean
  Compare To Constant8 : simulink/Logic and Bit Operations/Compare To Constant  relop=>=  const=80  OutDataTypeStr=boolean
  Demux : Demux  Outputs=3
  Logical Operator : Logic  Inputs=3  AllPortsSameDT=off  OutDataTypeStr=boolean
  Logical Operator1 : Logic  Operator=OR  Inputs=4  AllPortsSameDT=off  OutDataTypeStr=boolean
  Logical Operator2 : Logic  Operator=NOT  AllPortsSameDT=off  OutDataTypeStr=boolean
  Logical Operator3 : Logic  Operator=NOT  AllPortsSameDT=off  OutDataTypeStr=boolean
  Logical Operator4 : Logic  Operator=NOT  AllPortsSameDT=off  OutDataTypeStr=boolean
  Logical Operator5 : Logic  Operator=OR  AllPortsSameDT=off  OutDataTypeStr=boolean
  R2D : simulink_extras/Transformations/Radians to Degrees
  Vz : Selector  InputPortWidth=3  IndexOptions=Index vector (dialog)  Indices=3  OutputSizes=1
  pitch : Selector  InputPortWidth=3  IndexOptions=Index vector (dialog)  Indices=2  OutputSizes=1
  roll : Selector  InputPortWidth=3  IndexOptions=Index vector (dialog)  Indices=1  OutputSizes=1
  wires:
  Demux/1 -> Abs/1
  Compare To Constant/1 -> Logical Operator1/1
  Vz/1 -> Compare To Constant4/1
  Demux/3 -> Compare To Constant3/1, Compare To Constant2/1
  Compare To Constant3/1 -> Logical Operator/1
  Abs/1 -> Compare To Constant/1
  [Xe] -> Demux/1
  Compare To Constant1/1 -> Logical Operator1/2
  Abs1/1 -> Compare To Constant1/1
  Logical Operator1/1 -> Logical Operator2/1
  Demux/2 -> Abs1/1
  Logical Operator/1 -> Logical Operator1/4
  Compare To Constant2/1 -> Logical Operator1/3
  Compare To Constant4/1 -> Logical Operator/2
  [Ve] -> Vz/1
  [z_des] -> Compare To Constant5/1
  Compare To Constant5/1 -> Logical Operator/3
  [V_bat] -> Compare To Constant6/1
  Compare To Constant6/1 -> Logical Operator3/1
  Logical Operator2/1 -> Assertion1/1
  Logical Operator3/1 -> Assertion/1
  [Euler] -> R2D/1
  R2D/1 -> roll/1, pitch/1
  roll/1 -> Abs2/1
  Abs2/1 -> Compare To Constant7/1
  Logical Operator4/1 -> Assertion2/1
  Abs3/1 -> Compare To Constant8/1
  pitch/1 -> Abs3/1
  Logical Operator5/1 -> Logical Operator4/1
  Compare To Constant7/1 -> Logical Operator5/1
  Compare To Constant8/1 -> Logical Operator5/2

== system Marine_LocoMotive_UAV/Subsystem ==

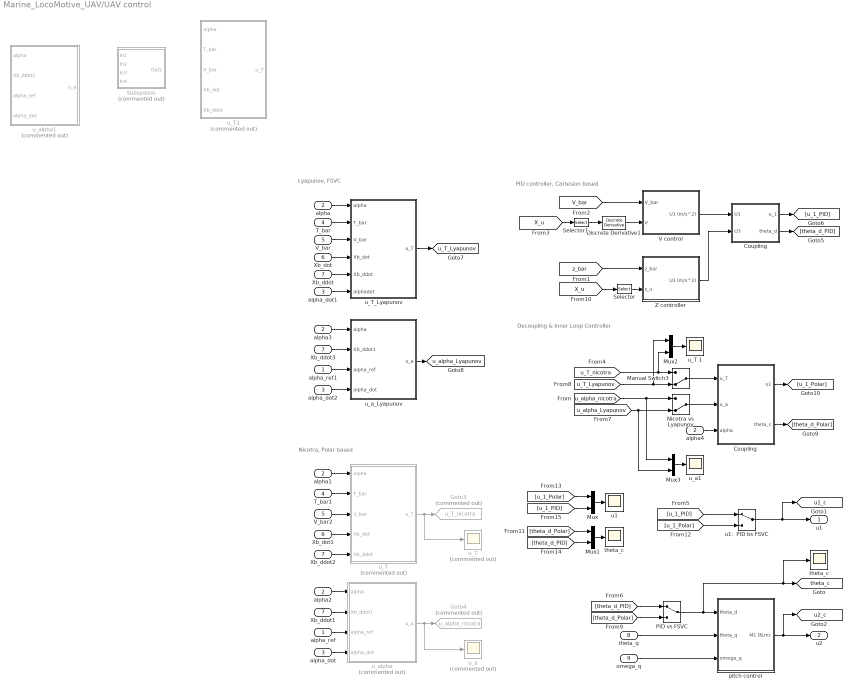
== system Marine_LocoMotive_UAV/UAV control ==
  note: Decoupling & Inner Loop Controller
  note: Lyapunov, FSVC
  note: Nicotra, Polar based
  note: PID controller, Cartesian based
  alpha_ref : Inport
  alpha : Inport  Port=2
  alpha_dot : Inport  Port=3
  T_bar : Inport  Port=4
  V_bar : Inport  Port=5
  Xb_dot : Inport  Port=6
  Xb_ddot : Inport  Port=7
  theta_q : Inport  Port=8
  omega_q : Inport  Port=9
  " theta_c " : Scope
  " u1 " : Scope
  Coupling : Subsystem
  "Coupling " : Subsystem
  Discrete Derivative1 : simulink/Discrete/Discrete Derivative  gainval=1.0  ICPrevScaledInput=0.0  OutMin=[]  OutMax=[]  OutDataType=fixdt(1, 16)  OutScaling=2^-10  DoSatur=off
  Goto3 : Goto  Commented=on  GotoTag=u_T_nicotra  TagVisibility=global
  Goto4 : Goto  Commented=on  GotoTag=u_alpha_nicotra  TagVisibility=global
  Manual Switch3 : ManualSwitch  CurrentSetting=0
  Mux{,1..3} (4 alike) : Mux  Inputs=2
  "Nicotra vs Lyapunov " : ManualSwitch  CurrentSetting=0
  PID vs FSVC : ManualSwitch
  Selector : Selector  InputPortWidth=2  IndexOptions=Index vector (dialog)  Indices=2  OutputSizes=1
  Selector1 : Selector  InputPortWidth=2  IndexOptions=Index vector (dialog)  Indices=1  OutputSizes=1
  Subsystem : Subsystem  Commented=on
  T_bar1 : InportShadow  Port=4
  V control : Subsystem
  V_bar2 : InportShadow  Port=5
  Xb_ddot1 : InportShadow  Port=7
  Xb_ddot2 : InportShadow  Port=7
  Xb_ddot3 : InportShadow  Port=7
  Xb_dot1 : InportShadow  Port=6
  Z controller : Subsystem
  alpha{1..4} (4 alike) : InportShadow  Port=2
  alpha_dot1 : InportShadow  Port=3
  alpha_dot2 : InportShadow  Port=3
  alpha_ref1 : InportShadow
  pitch control : Subsystem
  "theta_c " : Scope
  u1:  PID bs FSVC : ManualSwitch
  u_T : Subsystem  Commented=on
  "u_T " : Scope  Commented=on
  u_T 1 : Scope
  u_T1 : Subsystem  Commented=on
  u_T_Lyapunov : Subsystem
  u_a : Scope  Commented=on
  u_a1 : Scope
  u_a_Lyapunov : Subsystem
  u_alpha : Subsystem  Commented=on
  u_alpha1 : Subsystem  Commented=on
  u1 : Outport
  u2 : Outport  Port=2
  tag scope: theta_c=global, u1_c=global, u2_c=global, u_T_Lyapunov=global, u_alpha_Lyapunov=global
  wires:
  theta_q/1 -> pitch control/2(theta_q)
  omega_q/1 -> pitch control/3(omega_q)
  pitch control/1(M1 (N.m)) -> [u2_c], u2/1
  alpha4/1 -> "Coupling "/3(alpha)
  PID vs FSVC/1 -> " theta_c "/1, [theta_c], pitch control/1(theta_d)
  u1:  PID bs FSVC/1 -> [u1_c], u1/1
  [u_T_nicotra] -> Manual Switch3/1, Mux2/2
  alpha1/1 -> u_T/1(alpha)
  T_bar1/1 -> u_T/2(T_bar)
  V_bar2/1 -> u_T/3(V_bar)
  Xb_dot1/1 -> u_T/4(Xb_dot)
  Xb_ddot2/1 -> u_T/5(Xb_ddot)
  alpha2/1 -> u_alpha/1(alpha)
  Xb_ddot1/1 -> u_alpha/2(Xb_ddot1)
  alpha_ref/1 -> u_alpha/3(alpha_ref)
  alpha_dot/1 -> u_alpha/4("alpha_dot ")
  [z_bar] -> Z controller/1(z_bar)
  Selector/1 -> Z controller/2(z_u)
  [X_u] -> Selector/1
  [V_bar] -> V control/1(V_bar)
  [X_u] -> Selector1/1
  Discrete Derivative1/1 -> V control/2(V)
  Selector1/1 -> Discrete Derivative1/1
  V control/1(U1 (m/s^2)) -> Coupling/1(U1)
  Z controller/1(U3 (m/s^2)) -> Coupling/2(U3)
  Mux/1 -> " u1 "/1
  [u_1_PID] -> u1:  PID bs FSVC/1
  Mux1/1 -> "theta_c "/1
  [u_1_Polar] -> u1:  PID bs FSVC/2
  [u_T_Lyapunov] -> Manual Switch3/2, Mux2/1
  Mux2/1 -> u_T 1/1
  [u_alpha_Lyapunov] -> "Nicotra vs Lyapunov "/2, Mux3/2
  Mux3/1 -> u_a1/1
  [u_alpha_nicotra] -> "Nicotra vs Lyapunov "/1, Mux3/1
  "Nicotra vs Lyapunov "/1 -> "Coupling "/2(u_a)
  Manual Switch3/1 -> "Coupling "/1(u_T)
  [theta_d_PID] -> PID vs FSVC/1
  alpha/1 -> u_T_Lyapunov/1(alpha)
  T_bar/1 -> u_T_Lyapunov/2(T_bar)
  V_bar/1 -> u_T_Lyapunov/3(V_bar)
  Xb_dot/1 -> u_T_Lyapunov/4(Xb_dot)
  Xb_ddot/1 -> u_T_Lyapunov/5(Xb_ddot)
  alpha_dot1/1 -> u_T_Lyapunov/6(alphadot)
  alpha3/1 -> u_a_Lyapunov/1(alpha)
  Xb_ddot3/1 -> u_a_Lyapunov/2(Xb_ddot1)
  alpha_ref1/1 -> u_a_Lyapunov/3(alpha_ref)
  alpha_dot2/1 -> u_a_Lyapunov/4("alpha_dot ")
  u_alpha/1(u_a) -> u_a/1, Goto4/1
  Coupling/1(u_1) -> [u_1_PID]
  Coupling/2(theta_d) -> [theta_d_PID]
  u_T/1(u_T) -> "u_T "/1, Goto3/1
  u_a_Lyapunov/1(u_a) -> [u_alpha_Lyapunov]
  u_T_Lyapunov/1(u_T) -> [u_T_Lyapunov]
  [theta_d_Polar] -> PID vs FSVC/2
  "Coupling "/2(theta_c) -> [theta_d_Polar]
  [theta_d_Polar] -> Mux1/1
  "Coupling "/1(u1) -> [u_1_Polar]
  [u_1_Polar] -> Mux/1
  [theta_d_PID] -> Mux1/2
  [u_1_PID] -> Mux/2
